simulink model "SatElectricalSubsystemModel"  (R2023a)
settings: Solver=VariableStepAuto  StartTime=0.0  StopTime=14410  RelTol=1e-3
libraries: fl_lib x16, nesl_utility x11, ee_lib x10, batteryecm_lib x1
settings Model: PacingRate=1000  Creator=hrans  LastModifiedBy=hrans

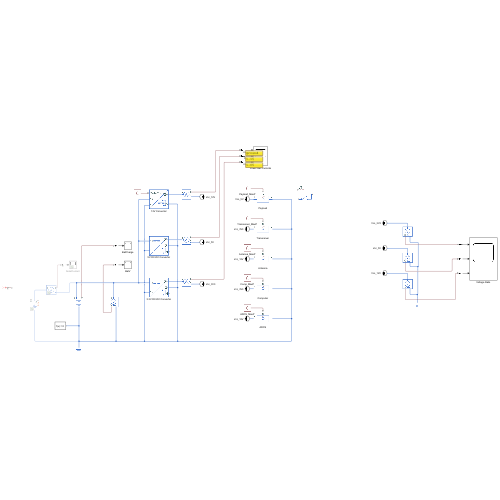
[thumbnail: Simulink's stored preview of the top-level diagram]
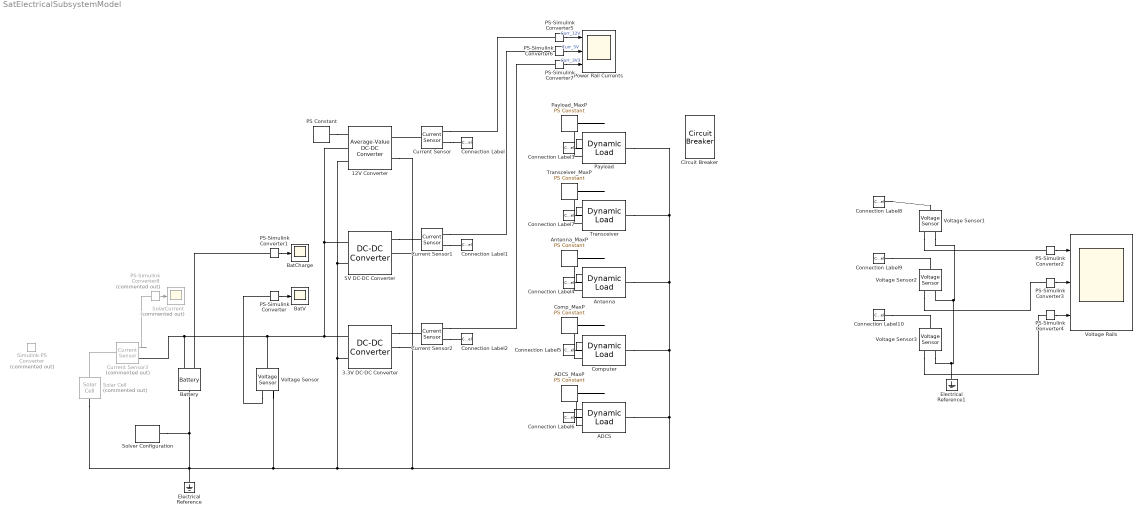
== system SatElectricalSubsystemModel ==
  12V Converter : ee_lib/Semiconductors & Converters/Converters/Average-Value DC-DC Converter  control_option=ee.enum.converters.controlinput.dutycycle  converter_type=ee.enum.converters.dcdctype.buck  efficiency_option=ee.enum.converters.efficiency.constant  efficiency_fixed=100  i_vec=[0, 2, 5] A  efficiency_vec=[90, 95, 98]
      settings: InternalSimscapePortConfiguration="{\"Bottom\":[],\"Left\":[{\"id\":\"DutyCycle\",\"label\":\"DutyCycle\",\"type\":\"input\"},{\"id\":\"p1\",\"label\":\"1+\",\"type\":\"foundation.electrical.electrical\"},{\"id\":\"n1\",\"label\":\"1-\",\"type\":\"foundation.electrical.electrical\"}],\"Right\":[{\"id\":\"p2\",\"label\":\"2+\",\"type\":\"foundation.electrical.electrical\"},{\"id\":\"n2\",\"label\":\"2-\",\"type\":\"foundation.electrical.electrical\"}],\"Top\":[]}"
  3.3V DC-DC Converter : ee_lib/Semiconductors & Converters/Converters/DC-DC Converter  Vref_option=ee.enum.converters.voltageref.internal  v_ref=3.3 V  P_rated=36 W  droop_enabled=false  droop_param=ee.enum.converters.droop.value  droop=0.1 V/A  droop_percent=2  Vref_droop=10 V  reversible=ee.enum.converters.directionality.unidirectional  G_diode=1e-8 1/Ohm  P_fixed=1 W  losses_option=ee.enum.converters.lossesOption.proportionalToSquaredCurrent  eff_rated=85  tableOption=ee.enum.converters.lossTableOptionThermal.currentTemp  i_eff_vec=[-2, -1, 1, 2] A  v_eff_vec=[15, 30, 45] V  eff_vec=[66, 76, 80, 74]  eff_2D_table=[66, 66, 66; 76, 76, 76; 80, 80, 80; 74, 74, 74]  model_dynamics=ee.enum.converters.dynamics.no  tau=0.02 s  v_ini=10 V  v1_min=1 V  R1=1000 Ohm  R2=1000 Ohm  enable_fault=simscape.enum.onoff.off  fault_condition=ee.enum.faults.faultInputCondition.greaterThan  fault_threshold=0.5  T_eff_vec=[280, 300, 320] K  eff_3D_table=repmat([66; 76; 80; 74], 1, 3, 3)  thermal_mass=100 J/K  initial_temperature=298.15 K
      settings: InternalSimscapePortConfiguration="{\"Bottom\":[],\"Left\":[{\"id\":\"p1\",\"label\":\"1+\",\"type\":\"foundation.electrical.electrical\"},{\"id\":\"n1\",\"label\":\"1-\",\"type\":\"foundation.electrical.electrical\"}],\"Right\":[{\"id\":\"p2\",\"label\":\"2+\",\"type\":\"foundation.electrical.electrical\"},{\"id\":\"n2\",\"label\":\"2-\",\"type\":\"foundation.electrical.electrical\"},{\"id\":\"H\",\"label\":\"H\",\"type\":\"foundation.thermal.thermal\"}],\"Top\":[]}"
  5V DC-DC Converter : ee_lib/Semiconductors & Converters/Converters/DC-DC Converter  Vref_option=ee.enum.converters.voltageref.internal  v_ref=5 V  P_rated=40 W  droop_enabled=false  droop_param=ee.enum.converters.droop.value  droop=0.1 V/A  droop_percent=2  Vref_droop=10 V  reversible=ee.enum.converters.directionality.unidirectional  G_diode=1e-8 1/Ohm  P_fixed=1 W  losses_option=ee.enum.converters.lossesOption.proportionalToSquaredCurrent  eff_rated=88  tableOption=ee.enum.converters.lossTableOptionThermal.currentTemp  i_eff_vec=[-2, -1, 1, 2] A  v_eff_vec=[15, 30, 45] V  eff_vec=[66, 76, 80, 74]  eff_2D_table=[66, 66, 66; 76, 76, 76; 80, 80, 80; 74, 74, 74]  model_dynamics=ee.enum.converters.dynamics.no  tau=0.02 s  v_ini=10 V  v1_min=1 V  R1=1000 Ohm  R2=1000 Ohm  enable_fault=simscape.enum.onoff.off  fault_condition=ee.enum.faults.faultInputCondition.greaterThan  fault_threshold=0.5  T_eff_vec=[280, 300, 320] K  eff_3D_table=repmat([66; 76; 80; 74], 1, 3, 3)  thermal_mass=100 J/K  initial_temperature=298.15 K
      settings: InternalSimscapePortConfiguration="{\"Bottom\":[],\"Left\":[{\"id\":\"p1\",\"label\":\"1+\",\"type\":\"foundation.electrical.electrical\"},{\"id\":\"n1\",\"label\":\"1-\",\"type\":\"foundation.electrical.electrical\"}],\"Right\":[{\"id\":\"p2\",\"label\":\"2+\",\"type\":\"foundation.electrical.electrical\"},{\"id\":\"n2\",\"label\":\"2-\",\"type\":\"foundation.electrical.electrical\"},{\"id\":\"H\",\"label\":\"H\",\"type\":\"foundation.thermal.thermal\"}],\"Top\":[]}"
  ADCS : ee_lib/Passive/Dynamic Load  load_type=ee.enum.dc_ac.dc  min_supply_voltage=11.5 V  pow_min=1 W  G_reverse=1e-6 S  deltaV=1e-3 V  f0=60 Hz  Vrms_min=200 V  Pmin=1e-3 W  enable_fault=simscape.enum.onoff.off  fault_action=simscape.enum.assert.action.none  t_fault=1 s  open_conductance=1e-4 S
      settings: InternalSimscapePortConfiguration="{\"Bottom\":[],\"Left\":[{\"id\":\"p\",\"label\":\"+\",\"type\":\"foundation.electrical.electrical\"}],\"Right\":[{\"id\":\"n\",\"label\":\"-\",\"type\":\"foundation.electrical.electrical\"}],\"Top\":[{\"id\":\"P\",\"label\":\"P\",\"type\":\"input\"}]}"
  ADCS_MaxP : fl_lib/Physical Signals/Sources/PS Constant  constant=7 W
  Antenna : ee_lib/Passive/Dynamic Load  load_type=ee.enum.dc_ac.dc  min_supply_voltage=8 V  pow_min=1 W  G_reverse=1e-6 S  deltaV=1e-3 V  f0=60 Hz  Vrms_min=200 V  Pmin=1e-3 W  enable_fault=simscape.enum.onoff.off  fault_action=simscape.enum.assert.action.none  t_fault=1 s  open_conductance=1e-4 S
      settings: InternalSimscapePortConfiguration="{\"Bottom\":[],\"Left\":[{\"id\":\"p\",\"label\":\"+\",\"type\":\"foundation.electrical.electrical\"}],\"Right\":[{\"id\":\"n\",\"label\":\"-\",\"type\":\"foundation.electrical.electrical\"}],\"Top\":[{\"id\":\"P\",\"label\":\"P\",\"type\":\"input\"}]}"
  Antenna_MaxP : fl_lib/Physical Signals/Sources/PS Constant  constant=11.00 W
  BatCharge : Scope
  BatV : Scope
  Battery : batteryecm_lib/Battery  Vnom=8.4 V  prm_dir=simscape.enum.battery.prm_dir.disabled  R1_dis=1 Ohm  R1_ch=1 Ohm  R1=2 Ohm  prm_AH=simscape.enum.battery.prm_AH.finite  AH=6.667 A*hr  V1=3.2 V  AH1=1 A*hr  prm_R2=simscape.enum.battery.prm_R2.disabled  R2=2000 Ohm  Tmeas=298.15 K  charge_measurement_port=simscape.enum.battery.enable.yes  prm_dyn=simscape.enum.battery.prm_dyn.rc1  Rp1=0.005 Ohm  tau1=30 s  Rp2=0.005 Ohm  tau2=30 s  Rp3=0.005 Ohm  tau3=30 s  Rp4=0.005 Ohm  tau4=30 s  Rp5=0.005 Ohm  tau5=30 s  prm_fade=simscape.enum.battery.prm_fade.disabled  N_fade=100  AH_fade=45 A*hr  R1_fade=2.02 Ohm  R1_ch_fade=2.02 Ohm  V1_fade=10.35 V  prm_age=simscape.enum.battery.prm_age.disabled  prm_age_OCV=simscape.enum.battery.prm_age_OCV.OCV  OCV_age=0.9  SOC_age=60  Tmeas_age=298.15 K  delta_time_age_vec=[0] d  temperature_age_vec=[273] K  OCV_scaling_age=2.2134e6  OCV_offset_age=1.632e6  temp_exp_age=0.515833569 V  t_exp_age=0.75  Vnom_T2=8.4 V  R1_T2=0.0015 Ohm  R1_T2_dis=2.2 Ohm  R1_T2_ch=2.2 Ohm  V1_T2=8.2 V  R2_T2=2200 Ohm  Rp1_T2=0.005 Ohm  tau1_T2=30 s  Rp2_T2=0.005 Ohm  tau2_T2=30 s  Rp3_T2=0.005 Ohm  tau3_T2=30 s  Rp4_T2=0.005 Ohm  tau4_T2=30 s  Rp5_T2=0.005 Ohm  tau5_T2=30 s  Tmeas2=273.15 K  thermal_port=simscape.enum.thermaleffects.omit  thermal_mass=30000 J/K  i_specify=off  i_priority=None  i=0 A  i_nominal_specify=off  i_nominal_unit=A  i_nominal_value=1  v_specify=off  v_priority=None  v=8.4 V  v_nominal_specify=on  v_nominal_unit=V  v_nominal_value=8.4  charge_specify=off  charge_priority=High  charge=50 A*hr  charge_nominal_specify=off  charge_nominal_unit=A*hr  charge_nominal_value=1  num_cycles_specify=off  num_cycles_priority=High  num_cycles=0  num_cycles_nominal_specify=off  num_cycles_nominal_unit=1  num_cycles_nominal_value=1  temperature_specify=off  temperature_priority=High  temperature=298.15 K  temperature_nominal_specify=off  temperature_nominal_unit=K  temperature_nominal_value=1
      settings: InternalSimscapePortConfiguration="{\"Bottom\":[],\"Left\":[{\"id\":\"p\",\"label\":\"+\",\"type\":\"foundation.electrical.electrical\"},{\"id\":\"q\",\"label\":\"q\",\"type\":\"output\"}],\"Right\":[{\"id\":\"n\",\"label\":\"-\",\"type\":\"foundation.electrical.electrical\"}],\"Top\":[]}"
  Circuit Breaker : ee_lib/Switches & Breakers/Circuit Breaker  R_closed=0.00001 mOhm  G_open=1e-6 1/Ohm  threshold=0.5 V  breaker_behavior=ee.enum.switches.breakerBehavior.zeroCrossingEnable
      settings: InternalSimscapePortConfiguration="{\"Bottom\":[],\"Left\":[{\"id\":\"vT\",\"label\":\"vT\",\"type\":\"input\"},{\"id\":\"p1\",\"label\":\"\",\"type\":\"foundation.electrical.electrical\"}],\"Right\":[{\"id\":\"p2\",\"label\":\"\",\"type\":\"foundation.electrical.electrical\"}],\"Top\":[]}"
  Comp_MaxP : fl_lib/Physical Signals/Sources/PS Constant  constant=2.31 W
  Computer : ee_lib/Passive/Dynamic Load  load_type=ee.enum.dc_ac.dc  min_supply_voltage=3.0 V  pow_min=1 W  G_reverse=1e-6 S  deltaV=1e-3 V  f0=60 Hz  Vrms_min=200 V  Pmin=1e-3 W  enable_fault=simscape.enum.onoff.off  fault_action=simscape.enum.assert.action.none  t_fault=1 s  open_conductance=1e-4 S
      settings: InternalSimscapePortConfiguration="{\"Bottom\":[],\"Left\":[{\"id\":\"p\",\"label\":\"+\",\"type\":\"foundation.electrical.electrical\"}],\"Right\":[{\"id\":\"n\",\"label\":\"-\",\"type\":\"foundation.electrical.electrical\"}],\"Top\":[{\"id\":\"P\",\"label\":\"P\",\"type\":\"input\"}]}"
  Connection Label{,4,6,10} (4 alike) : ConnectionLabel  Label=Vcc_12V
  Connection Label1 : ConnectionLabel  Label=Vcc_5V
  Connection Label{2,5,7..8} (4 alike) : ConnectionLabel  Label=Vcc_3V3
  Connection Label3 : ConnectionLabel  Label=Vcc_5V
  Connection Label9 : ConnectionLabel  Label=Vcc_5V
  Current Sensor : fl_lib/Electrical/Electrical Sensors/Current Sensor
  Current Sensor1 : fl_lib/Electrical/Electrical Sensors/Current Sensor
  Current Sensor2 : fl_lib/Electrical/Electrical Sensors/Current Sensor
  Current Sensor3 : fl_lib/Electrical/Electrical Sensors/Current Sensor  Commented=on
  Electrical Reference : fl_lib/Electrical/Electrical Elements/Electrical Reference
  Electrical Reference1 : fl_lib/Electrical/Electrical Elements/Electrical Reference
  PS Constant : fl_lib/Physical Signals/Sources/PS Constant  constant=1
  PS-Simulink Converter{,1..7} (8 alike) : nesl_utility/PS-Simulink Converter  PhysicalDomain=network_engine_domain  SubClassName=ps_output  LeftPortType=input  RightPortType=output  PseudoPeriodic=off  Frequencies=[]  VectorFormat=inherit  Unit=inherit  AffineConversion=off
  PS-Simulink Converter8 : nesl_utility/PS-Simulink Converter  Commented=on  PhysicalDomain=network_engine_domain  SubClassName=ps_output  LeftPortType=input  RightPortType=output  PseudoPeriodic=off  Frequencies=[]  VectorFormat=inherit  Unit=inherit  AffineConversion=off
  Payload : ee_lib/Passive/Dynamic Load  load_type=ee.enum.dc_ac.dc  min_supply_voltage=4.5 V  pow_min=1 W  G_reverse=1e-6 S  deltaV=1e-3 V  f0=60 Hz  Vrms_min=200 V  Pmin=1e-3 W  enable_fault=simscape.enum.onoff.off  fault_action=simscape.enum.assert.action.none  t_fault=1 s  open_conductance=1e-4 S
      settings: InternalSimscapePortConfiguration="{\"Bottom\":[],\"Left\":[{\"id\":\"p\",\"label\":\"+\",\"type\":\"foundation.electrical.electrical\"}],\"Right\":[{\"id\":\"n\",\"label\":\"-\",\"type\":\"foundation.electrical.electrical\"}],\"Top\":[{\"id\":\"P\",\"label\":\"P\",\"type\":\"input\"}]}"
  Payload_MaxP : fl_lib/Physical Signals/Sources/PS Constant  constant=11.55 W
  Power Rail Currents : Scope  NumInputPorts=3
  Simulink-PS Converter : nesl_utility/Simulink-PS Converter  Commented=on  PhysicalDomain=network_engine_domain  SubClassName=ps_input  LeftPortType=input  RightPortType=output  PseudoPeriodic=off  Frequencies=[]  NoiseDistribution=none  NoiseParameters=[]  Unit=W/m^2  AffineConversion=on  FilteringAndDerivatives=provide  SimscapeFilterOrder=1  InputFilterTimeConstant=0.001  UdotUserProvided=0
  Solar Cell : ee_lib/Sources/Solar Cell  Commented=on  prm=1  Isc=2.07 A  Voc=10.76 V  Is=1e-6 A  Is2=0 A  Iph=7.34 A  Ir0=1339.6 W/m^2  ec=1.5  N2=2  Rs=0 Ohm  Rp=inf Ohm  N_series=4  N_parallel=4  TIPH1=0 1/K  EG=1.11 eV  TXIS1=3  TXIS2=3  TRS1=0  TRP1=0  Tmeas=25 degC  TFIXED=25 degC  thermal_mass=100 J/K  initial_temperature=25 degC
      settings: InternalSimscapePortConfiguration="{\"Bottom\":[],\"Left\":[{\"id\":\"Ir\",\"label\":\"Ir\",\"type\":\"input\"},{\"id\":\"p\",\"label\":\"+\",\"type\":\"foundation.electrical.electrical\"},{\"id\":\"H\",\"label\":\"H\",\"type\":\"foundation.thermal.thermal\"}],\"Right\":[{\"id\":\"n\",\"label\":\"-\",\"type\":\"foundation.electrical.electrical\"}],\"Top\":[]}"
  SolarCurrent : Scope  Commented=on
  Solver Configuration : nesl_utility/Solver Configuration  PhysicalDomain=network_engine_domain  SubClassName=solver  LeftPortType=input  RightPortType=generic  Tones=[]  Harmonics=[]  SimulateNoise=off  Profile=off  UseLocalSampling=off  EnableSwitchedLinearOptims=on  FrequencyDomain=off  UseCCode=off  RelTol=0.001  AbsTol=0.001  MinStep=1e-09  ToWorkspace=off  RevertToSquareIcSolve=off  NumHomotopyIterations=100  PhasorMode=off  PhasorModeNumHarmonics=1  ConsistencySolver=NEWTON_XTOL_AFTER_FTOL  IndexReductionMethod=DerivativeReplacement  DoDC=on  ResidualTolerance=1e-09  ConsistencyTolSource=GLOBAL  ConsistencyAbsTol=0.001  ConsistencyRelTol=0.001  ConsistencyTolFactor=0.001  UseLocalSolver=on  LocalSolverChoice=NE_BACKWARD_EULER_ADVANCER  ResolveIndetEquations=on  FunctionEvalNumThread=1  LocalSolverSampleTime=0.001  DoFixedCost=on  MaxNonlinIter=3  MaxModeIter=2  ComputeImpulses=off  ImpulseIterations=2  LinearAlgebra=auto  LinearAlgebraNumThread=0  EquationFormulation=NE_TIME_EF  DelaysMemoryBudget=1024  AutomaticFiltering=on  FilteringTimeConstant=0.001  PartitionStorageMethod=AS_NEEDED  PartitionMemoryBudget=1024  PartitionMethod=ROBUST
  Transceiver : ee_lib/Passive/Dynamic Load  load_type=ee.enum.dc_ac.dc  min_supply_voltage=3.0 V  pow_min=1 W  G_reverse=1e-6 S  deltaV=1e-3 V  f0=60 Hz  Vrms_min=200 V  Pmin=1e-3 W  enable_fault=simscape.enum.onoff.off  fault_action=simscape.enum.assert.action.none  t_fault=1 s  open_conductance=1e-4 S
      settings: InternalSimscapePortConfiguration="{\"Bottom\":[],\"Left\":[{\"id\":\"p\",\"label\":\"+\",\"type\":\"foundation.electrical.electrical\"}],\"Right\":[{\"id\":\"n\",\"label\":\"-\",\"type\":\"foundation.electrical.electrical\"}],\"Top\":[{\"id\":\"P\",\"label\":\"P\",\"type\":\"input\"}]}"
  Transceiver_MaxP : fl_lib/Physical Signals/Sources/PS Constant  constant=14.4 W
  Voltage Rails : Scope  NumInputPorts=3
  Voltage Sensor{,1..3} (4 alike) : fl_lib/Electrical/Electrical Sensors/Voltage Sensor
  wires:
  ? -> Simulink-PS Converter/1
  PS-Simulink Converter2/1 -> Voltage Rails/1
  PS-Simulink Converter3/1 -> Voltage Rails/2
  PS-Simulink Converter4/1 -> Voltage Rails/3
  PS-Simulink Converter1/1 -> BatCharge/1
  PS-Simulink Converter/1 -> BatV/1
  PS-Simulink Converter5/1 -> Power Rail Currents/1  "Curr_12V"
  PS-Simulink Converter7/1 -> Power Rail Currents/3  "Curr_3V3"
  PS-Simulink Converter6/1 -> Power Rail Currents/2  "Curr_5V"
  PS-Simulink Converter8/1 -> SolarCurrent/1
  connections:
  Transceiver/RConn1 -- Solar Cell/RConn1 -- Electrical Reference/LConn1 -- Solver Configuration/RConn1 -- Battery/RConn1 -- Voltage Sensor/RConn2 -- 12V Converter/LConn3 -- 5V DC-DC Converter/LConn2 -- 3.3V DC-DC Converter/LConn2 -- 3.3V DC-DC Converter/RConn2 -- 12V Converter/RConn2 -- 5V DC-DC Converter/RConn2 -- ADCS/RConn1 -- Computer/RConn1 -- Antenna/RConn1 -- Payload/RConn1
  Current Sensor3/RConn2 -- 12V Converter/LConn2 -- 5V DC-DC Converter/LConn1 -- 3.3V DC-DC Converter/LConn1 -- Voltage Sensor/LConn1 -- Battery/LConn1
  Connection Label5/LConn1 -- Computer/LConn1
  Connection Label4/LConn1 -- Antenna/LConn1
  Connection Label7/LConn1 -- Transceiver/LConn1
  Antenna_MaxP/RConn1 -- Antenna/LConn2
  Battery/LConn2 -- PS-Simulink Converter1/LConn1
  Voltage Sensor/RConn1 -- PS-Simulink Converter/LConn1
  Connection Label3/LConn1 -- Payload/LConn1
  ADCS_MaxP/RConn1 -- ADCS/LConn2
  Comp_MaxP/RConn1 -- Computer/LConn2
  Connection Label6/LConn1 -- ADCS/LConn1
  Transceiver_MaxP/RConn1 -- Transceiver/LConn2
  Payload_MaxP/RConn1 -- Payload/LConn2
  Connection Label8/LConn1 -- Voltage Sensor1/LConn1
  Connection Label9/LConn1 -- Voltage Sensor2/LConn1
  Voltage Sensor1/RConn2 -- Electrical Reference1/LConn1 -- Voltage Sensor3/RConn2 -- Voltage Sensor2/RConn2
  Connection Label10/LConn1 -- Voltage Sensor3/LConn1
  Voltage Sensor1/RConn1 -- PS-Simulink Converter2/LConn1
  Voltage Sensor2/RConn1 -- PS-Simulink Converter3/LConn1
  Voltage Sensor3/RConn1 -- PS-Simulink Converter4/LConn1
  Current Sensor/LConn1 -- 12V Converter/RConn1
  Current Sensor/RConn2 -- Connection Label/LConn1
  5V DC-DC Converter/RConn1 -- Current Sensor1/LConn1
  Current Sensor1/RConn2 -- Connection Label1/LConn1
  Current Sensor2/RConn2 -- Connection Label2/LConn1
  3.3V DC-DC Converter/RConn1 -- Current Sensor2/LConn1
  Current Sensor/RConn1 -- PS-Simulink Converter5/LConn1
  Current Sensor1/RConn1 -- PS-Simulink Converter6/LConn1
  Current Sensor2/RConn1 -- PS-Simulink Converter7/LConn1
  Solar Cell/LConn2 -- Current Sensor3/LConn1
  Current Sensor3/RConn1 -- PS-Simulink Converter8/LConn1
  PS Constant/RConn1 -- 12V Converter/LConn1
